simulink model "SistemaPFSIRA"  (R2023a)
settings: Solver=ode45  StartTime=0.0  StopTime=10.0  MaxStep=1e-3  RelTol=1e-3
libraries: slpidlib x1
settings Model: Creator=Dell  LastModifiedBy=HP
settings DataIOCC: ReturnWorkspaceOutputs=off  TimeSaveName=t
settings DebuggingCC: AlgebraicLoopMsg=none  ArtificialAlgebraicLoopMsg=none  InheritedTsInSrcMsg=none

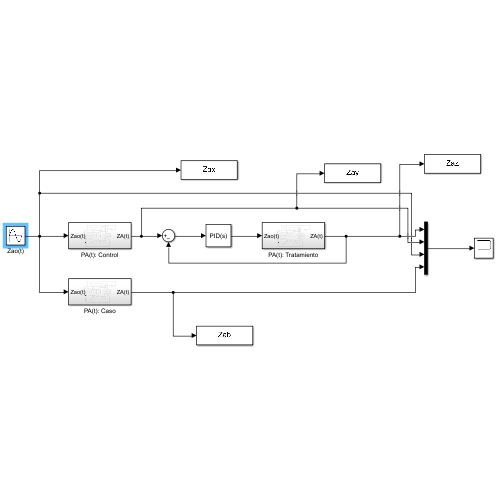
[thumbnail: Simulink's stored preview of the top-level diagram]
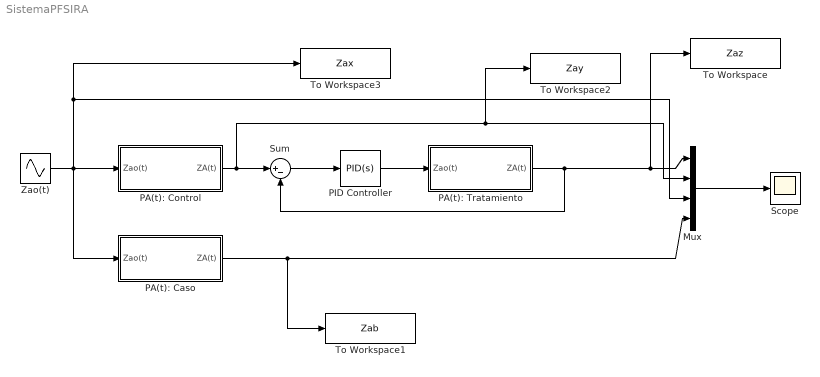
== system SistemaPFSIRA ==
  Mux : Mux
  PA(t): Caso : Subsystem
  PA(t): Control : Subsystem
  PA(t): Tratamiento : Subsystem
  PID Controller : slpidlib/PID Controller  Controller=PID  Form=Parallel  TimeDomain=Continuous-time  UseExternalTs=off  SampleTime=-1  IntegratorMethod=Forward Euler  FilterMethod=Forward Euler  ControllerParametersSource=internal  P=7504.3128  I=40028.7836  UseKiTs=off  D=312.5866  N=104491.5556  UseFilter=on  TunerSelectOption=Transfer Function Based (PID Tuner App)  InitialConditionSource=internal  InitialConditionForIntegrator=0  InitialConditionForFilter=0  DifferentiatorICPrevScaledInput=0  ExternalReset=none  TrackingMode=off  Kt=1  LimitOutput=off  SatLimitsSource=internal  UpperSaturationLimit=inf  LowerSaturationLimit=-inf  LinearizeAsGain=on  AntiWindupMode=none  Kb=1  LimitIntegrator=off  UpperIntegratorSaturationLimit=inf  LowerIntegratorSaturationLimit=-inf  POutMin=[]  POutMax=[]  IOutMin=[]  IOutMax=[]  DOutMin=[]  DOutMax=[]  NOutMin=[]  NOutMax=[]  SumOutMin=[]  SumOutMax=[]  SaturationOutMin=[]  SaturationOutMax=[]  PParamMin=[]  PParamMax=[]  IParamMin=[]  IParamMax=[]  DParamMin=[]  DParamMax=[]  NParamMin=[]  NParamMax=[]  KbParamMin=[]  KbParamMax=[]  KtParamMin=[]  KtParamMax=[]  KbOutMin=[]  KbOutMax=[]  KtOutMin=[]  KtOutMax=[]  IntegratorOutMin=[]  IntegratorOutMax=[]  FilterOutMin=[]  FilterOutMax=[]  SumI1OutMin=[]  SumI1OutMax=[]  SumI2OutMin=[]  SumI2OutMax=[]  SumI3OutMin=[]  SumI3OutMax=[]  SumI4OutMin=[]  SumI4OutMax=[]  SumDOutMin=[]  SumDOutMax=[]  DifferentiatorOutMin=[]  DifferentiatorOutMax=[]  FilterDiffOutCoefMin=[]  FilterDiffOutCoefMax=[]  ReciprocalOutMin=[]  ReciprocalOutMax=[]  SumDenOutMin=[]  SumDenOutMax=[]  SumNumOutMin=[]  SumNumOutMax=[]  DivideOutMin=[]  DivideOutMax=[]  UdiffTsProdOutMin=[]  UdiffTsProdOutMax=[]  NTsProdOutMin=[]  NTsProdOutMax=[]  UintegralTsProdOutMin=[]  UintegralTsProdOutMax=[]  UngainTsProdOutMin=[]  UngainTsProdOutMax=[]  ClampingZeroOutDataTypeStr=Inherit: Inherit via back propagation  ClampingZeroOutMin=[]  ClampingZeroOutMax=[]  FilterDenConstantOutDataTypeStr=Inherit: Inherit via back propagation  FilterDenConstantOutMin=[]  FilterDenConstantOutMax=[]  PCopyOutDataTypeStr=Inherit: Inherit via back propagation  PCopyOutMin=[]  PCopyOutMax=[]  NCopyOutDataTypeStr=Inherit: Inherit via back propagation  NCopyOutMin=[]  NCopyOutMax=[]  IntegratorContinuousStateAttributes=''  IntegratorStateMustResolveToSignalObject=off  IntegratorRTWStateStorageClass=Auto  FilterContinuousStateAttributes=''  FilterStateMustResolveToSignalObject=off  FilterRTWStateStorageClass=Auto  ParallelPVariant=InternalParameters  IdealPVariant=Disabled  IVariant=InternalParameters  DVariant=InternalParameters  IntegratorVariant=Continuous  SatVariant=Disabled  AWVariant=Passthrough  PCopyVariant=Disabled  TRVariant=Disabled  FdbkBlocksVariant=Forward  IdealPFdbkVariant=Disabled  SatFdbkVariant=Disabled  DerivativeFilterVariant=ContFilter  NVariant=InternalParameters  NCopyVariant=Disabled  FilterICVariant=InternalICsFilter  IntegratorICVariant=InternalICs  ExternalResetVariant=Disabled  TRSumVariant=Passthrough  SumFdbkVariant=Disabled  SumVariant=Sum_PID  TsampFilterVariant=InternalTs  TsampNgainVariant=Passthrough  TsampIntegralVariant=Disabled_SignalSpec  ExternalSaturationOutDataTypeStr=Inherit: Same as second input
  Scope : Scope
  Sum : Sum  Inputs=|+-
  To Workspace : ToWorkspace  VariableName=Zaz  SampleTime=-1
  To Workspace1 : ToWorkspace  VariableName=Zab  SampleTime=-1
  To Workspace2 : ToWorkspace  VariableName=Zay  SampleTime=-1
  To Workspace3 : ToWorkspace  VariableName=Zax  SampleTime=-1
  Zao(t) : Sin  Frequency=pi
  wires:
  Mux/1 -> Scope/1
  Sum/1 -> PID Controller/1
  PID Controller/1 -> PA(t): Tratamiento/1(Zao(t))
  PA(t): Tratamiento/1(ZA(t)) -> Sum/2, To Workspace/1, Mux/1
  PA(t): Control/1(ZA(t)) -> To Workspace2/1, Mux/2, Sum/1
  Zao(t)/1 -> PA(t): Caso/1(Zao(t)), To Workspace3/1, Mux/3, PA(t): Control/1(Zao(t))
  PA(t): Caso/1(ZA(t)) -> To Workspace1/1, Mux/4

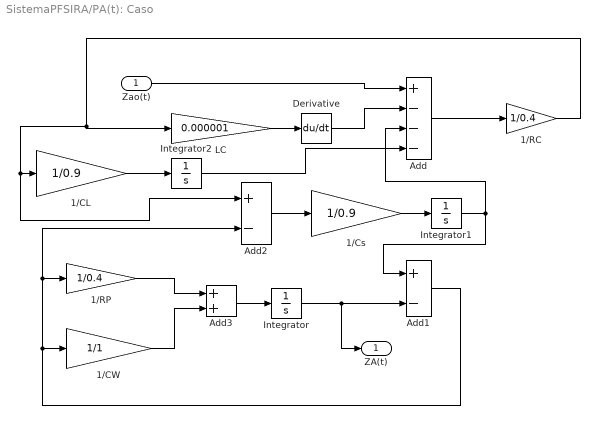
== system SistemaPFSIRA/PA(t): Caso ==
  Zao(t) : Inport
  1/CL : Gain  Gain=1/0.9
  1/CW : Gain  Gain=1/1
  1/Cs : Gain  Gain=1/0.9
  1/RC : Gain  Gain=1/0.4
  1/RP : Gain  Gain=1/0.4
  Add : Sum  Inputs=+---
  Add1 : Sum  Inputs=+-
  Add2 : Sum  Inputs=+-
  Add3 : Sum
  Derivative : Derivative
  Integrator : Integrator
  Integrator1 : Integrator
  Integrator2 : Integrator
  LC : Gain  Gain=0.000001
  ZA(t) : Outport
  wires:
  Add1/1 -> 1/CW/1, Add2/2, 1/RP/1
  1/CL/1 -> Integrator2/1
  1/CW/1 -> Add3/2
  LC/1 -> Derivative/1
  1/Cs/1 -> Integrator1/1
  1/RP/1 -> Add3/1
  Add2/1 -> 1/Cs/1
  1/RC/1 -> LC/1, Add2/1, 1/CL/1
  Integrator1/1 -> Add1/1, Add/3
  Add/1 -> 1/RC/1
  Integrator/1 -> ZA(t)/1, Add1/2
  Add3/1 -> Integrator/1
  Zao(t)/1 -> Add/1
  Derivative/1 -> Add/2
  Integrator2/1 -> Add/4

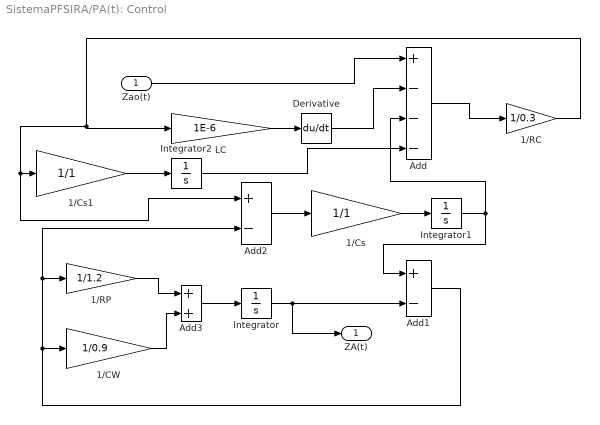
== system SistemaPFSIRA/PA(t): Control ==
  Zao(t) : Inport
  1/CW : Gain  Gain=1/0.9
  1/Cs : Gain  Gain=1/1
  1/Cs1 : Gain  Gain=1/1
  1/RC : Gain  Gain=1/0.3
  1/RP : Gain  Gain=1/1.2
  Add : Sum  Inputs=+---
  Add1 : Sum  Inputs=+-
  Add2 : Sum  Inputs=+-
  Add3 : Sum
  Derivative : Derivative
  Integrator : Integrator
  Integrator1 : Integrator
  Integrator2 : Integrator
  LC : Gain  Gain=1E-6
  ZA(t) : Outport
  wires:
  Zao(t)/1 -> Add/1
  Derivative/1 -> Add/2
  Add3/1 -> Integrator/1
  Integrator/1 -> ZA(t)/1, Add1/2
  LC/1 -> Derivative/1
  Add2/1 -> 1/Cs/1
  Add/1 -> 1/RC/1
  1/RC/1 -> LC/1, Add2/1, 1/Cs1/1
  1/Cs/1 -> Integrator1/1
  Integrator1/1 -> Add1/1, Add/3
  Add1/1 -> 1/CW/1, Add2/2, 1/RP/1
  1/RP/1 -> Add3/1
  1/CW/1 -> Add3/2
  1/Cs1/1 -> Integrator2/1
  Integrator2/1 -> Add/4

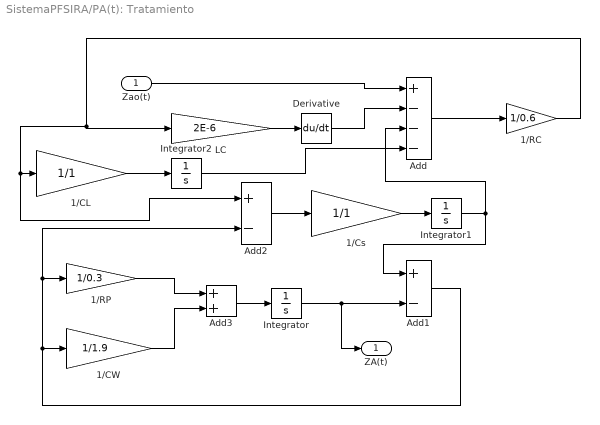
== system SistemaPFSIRA/PA(t): Tratamiento ==
  Zao(t) : Inport
  1/CL : Gain  Gain=1/1
  1/CW : Gain  Gain=1/1.9
  1/Cs : Gain  Gain=1/1
  1/RC : Gain  Gain=1/0.6
  1/RP : Gain  Gain=1/0.3
  Add : Sum  Inputs=+---
  Add1 : Sum  Inputs=+-
  Add2 : Sum  Inputs=+-
  Add3 : Sum
  Derivative : Derivative
  Integrator : Integrator
  Integrator1 : Integrator
  Integrator2 : Integrator
  LC : Gain  Gain=2E-6
  ZA(t) : Outport
  wires:
  Add1/1 -> 1/CW/1, Add2/2, 1/RP/1
  1/CL/1 -> Integrator2/1
  1/CW/1 -> Add3/2
  LC/1 -> Derivative/1
  1/Cs/1 -> Integrator1/1
  1/RP/1 -> Add3/1
  Add2/1 -> 1/Cs/1
  1/RC/1 -> LC/1, Add2/1, 1/CL/1
  Integrator1/1 -> Add1/1, Add/3
  Add/1 -> 1/RC/1
  Integrator/1 -> ZA(t)/1, Add1/2
  Add3/1 -> Integrator/1
  Zao(t)/1 -> Add/1
  Derivative/1 -> Add/2
  Integrator2/1 -> Add/4
